simulink model "WaterTankModel_ExternalController"  (Simulink 8.1)
settings: Solver=ode3  StartTime=0.0  StopTime=150.0  FixedStep=0.001  RelTol=1e-3
InitFcn:
  | initparametersDACADC
  | WT_SerialCom_Model
undefined symbols (not defined in the file): Ad, Bd, Cd, Dd, k0, k1, k2, SAMPLING_PERIOD, WT_CALIBRATION, x0, x_ref
libraries: GisooLib x7
settings Model: Creator=behdad  LastModifiedBy=behdad

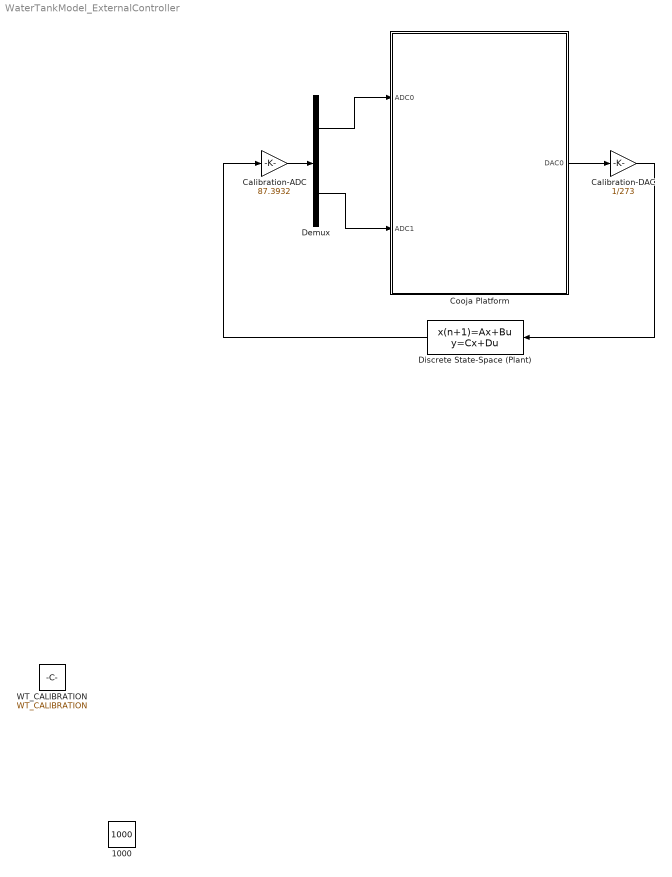
== system WaterTankModel_ExternalController ==
  1000 : Constant  Value=1000
  Calibration-ADC : Gain  Gain=87.3932
  Calibration-DAC : Gain  Gain=1/273
  Cooja Platform : Subsystem  AncestorBlock=GisooLib/Gisoo Platform  TreatAsAtomicUnit=on
  Demux : Demux  Outputs=2
  Discrete State-Space (Plant) : DiscreteStateSpace  A=Ad  B=Bd  C=Cd  D=Dd  X0=x0  SampleTime=-1
  WT_CALIBRATION : Constant  Value=WT_CALIBRATION
  wires:
  Discrete State-Space (Plant)/1 -> Calibration-ADC/1
  Cooja Platform/1(DAC0) -> Calibration-DAC/1
  Calibration-DAC/1 -> Discrete State-Space (Plant)/1
  Calibration-ADC/1 -> Demux/1
  Demux/1 -> Cooja Platform/1(ADC0)
  Demux/2 -> Cooja Platform/2(ADC1)

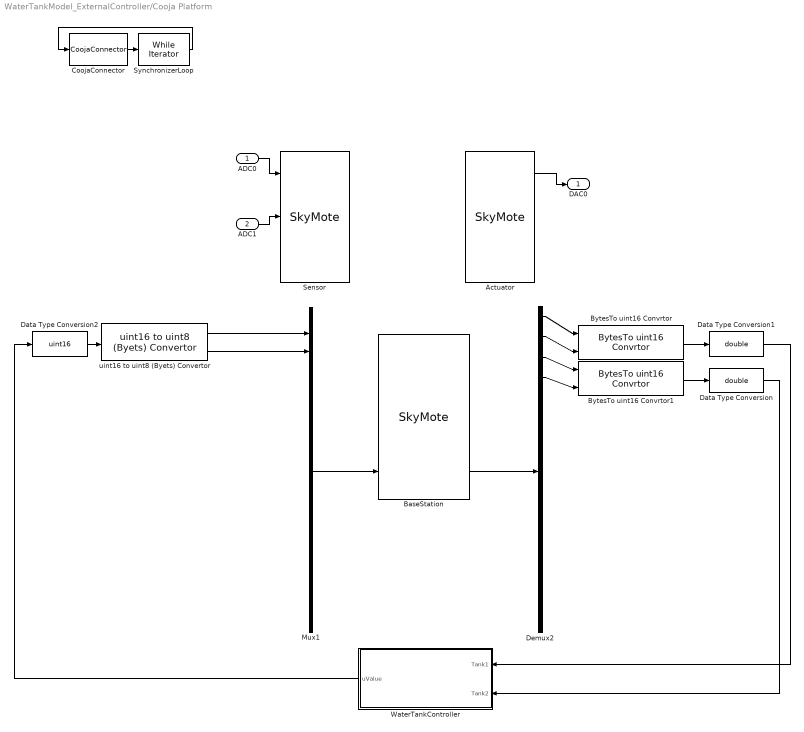
== system WaterTankModel_ExternalController/Cooja Platform ==
  ADC0 : Inport
  ADC1 : Inport  Port=2
  Actuator : GisooLib/SkyMote  moteID=4  PacketType=6
  BaseStation : GisooLib/SkyMote  moteID=3  PacketType=6
  BytesTo uint16 Convrtor : GisooLib/BytesTo uint16 Convrtor
  BytesTo uint16 Convrtor1 : GisooLib/BytesTo uint16 Convrtor
  CoojaConnector : GisooLib/Cooja Platform/CoojaConnector
      link override "Check that we don't loop forever, if Cooja never answers": const=30000
  Data Type Conversion : DataTypeConversion  OutDataTypeStr=double
  Data Type Conversion1 : DataTypeConversion  OutDataTypeStr=double
  Data Type Conversion2 : DataTypeConversion  OutDataTypeStr=uint16
  Demux2 : Demux  Outputs=16
  Mux1 : Mux  Inputs=16
  Sensor : GisooLib/SkyMote  moteID=1  PacketType=6
  SynchronizerLoop : WhileIterator  MaxIters=-1  WhileBlockType=do-while  ShowIterationPort=on
  WaterTankController : Subsystem
  uint16 to uint8 (Byets) Convertor : GisooLib/uint16 to uint8 (Byets) Convertor
  DAC0 : Outport
  wires:
  Actuator/1 -> DAC0/1
  ADC0/1 -> Sensor/1
  ADC1/1 -> Sensor/2
  SynchronizerLoop/1 -> CoojaConnector/1
  CoojaConnector/1 -> SynchronizerLoop/1
  BaseStation/3 -> Demux2/1
  Mux1/1 -> BaseStation/3
  uint16 to uint8 (Byets) Convertor/1 -> Mux1/1
  uint16 to uint8 (Byets) Convertor/2 -> Mux1/2
  Demux2/1 -> BytesTo uint16 Convrtor/1
  Demux2/2 -> BytesTo uint16 Convrtor/2
  BytesTo uint16 Convrtor/1 -> Data Type Conversion1/1
  BytesTo uint16 Convrtor1/1 -> Data Type Conversion/1
  Data Type Conversion2/1 -> uint16 to uint8 (Byets) Convertor/1
  Data Type Conversion/1 -> WaterTankController/2(Tank2)
  WaterTankController/1(uValue) -> Data Type Conversion2/1
  Demux2/3 -> BytesTo uint16 Convrtor1/1
  Demux2/4 -> BytesTo uint16 Convrtor1/2
  Data Type Conversion1/1 -> WaterTankController/1(Tank1)

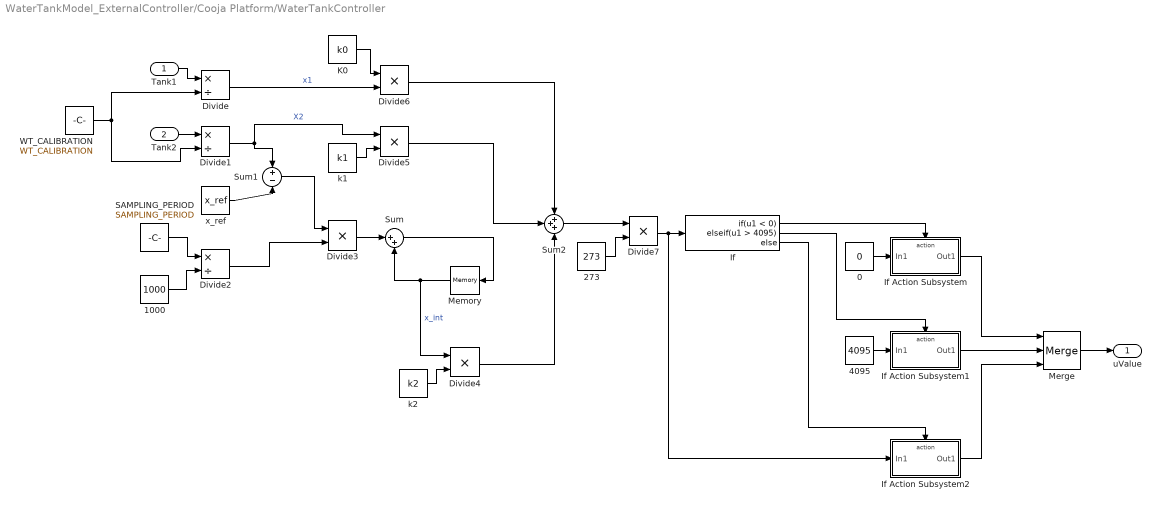
== system WaterTankModel_ExternalController/Cooja Platform/WaterTankController ==
  Tank1 : Inport
  Tank2 : Inport  Port=2
  0 : Constant  Value=0
  1000 : Constant  Value=1000
  273 : Constant  Value=273
  4095 : Constant  Value=4095
  Divide : Product  Inputs=*/
  Divide1 : Product  Inputs=*/
  Divide2 : Product  Inputs=*/
  Divide{3..7} (5 alike) : Product  Inputs=**
  If : If  IfExpression=u1 < 0  ElseIfExpressions=u1 > 4095
  If Action Subsystem : Subsystem  TreatAsAtomicUnit=on
  If Action Subsystem1 : Subsystem  TreatAsAtomicUnit=on
  If Action Subsystem2 : Subsystem  TreatAsAtomicUnit=on
  K0 : Constant  Value=k0
  Memory : Memory  InheritSampleTime=on
  Merge : Merge  Inputs=3
  SAMPLING_PERIOD : Constant  Value=SAMPLING_PERIOD
  Sum : Sum  Inputs=|++
  Sum1 : Sum  Inputs=+-
  Sum2 : Sum  Inputs=+++
  WT_CALIBRATION : Constant  Value=WT_CALIBRATION
  k1 : Constant  Value=k1
  k2 : Constant  Value=k2
  x_ref : Constant  Value=x_ref
  uValue : Outport
  wires:
  If Action Subsystem/1(Out1) -> Merge/1
  Divide5/1 -> Sum2/2
  0/1 -> If Action Subsystem/1(In1)
  1000/1 -> Divide2/2
  Divide2/1 -> Divide3/2
  x_ref/1 -> Sum1/2
  k1/1 -> Divide5/2
  Tank2/1 -> Divide1/1
  Divide1/1 -> Divide5/1, Sum1/1  "X2"
  Divide3/1 -> Sum/1
  Memory/1 -> Sum/2, Divide4/1  "x_int"
  WT_CALIBRATION/1 -> Divide/2, Divide1/2
  Divide/1 -> Divide6/2  "x1"
  k2/1 -> Divide4/2
  Tank1/1 -> Divide/1
  Divide6/1 -> Sum2/1
  If Action Subsystem2/1(Out1) -> Merge/3
  4095/1 -> If Action Subsystem1/1(In1)
  Sum2/1 -> Divide7/1
  Divide7/1 -> If/1, If Action Subsystem2/1(In1)
  If/3 -> If Action Subsystem2/Action
  If/1 -> If Action Subsystem/Action
  If Action Subsystem1/1(Out1) -> Merge/2
  Merge/1 -> uValue/1
  273/1 -> Divide7/2
  If/2 -> If Action Subsystem1/Action
  Sum/1 -> Memory/1
  Sum1/1 -> Divide3/1
  K0/1 -> Divide6/1
  Divide4/1 -> Sum2/3
  SAMPLING_PERIOD/1 -> Divide2/1

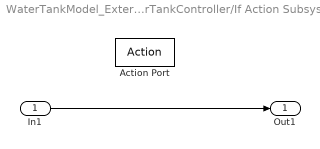
== system WaterTankModel_ExternalController/Cooja Platform/WaterTankController/If Action Subsystem ==
  In1 : Inport
  Action Port : ActionPort  ActionType=then
  Out1 : Outport
  wires:
  In1/1 -> Out1/1

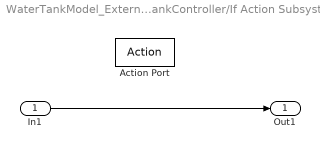
== system WaterTankModel_ExternalController/Cooja Platform/WaterTankController/If Action Subsystem1 ==
  In1 : Inport
  Action Port : ActionPort  ActionType=elseif
  Out1 : Outport
  wires:
  In1/1 -> Out1/1

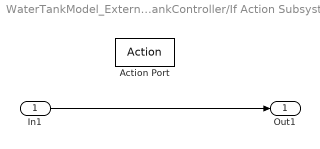
== system WaterTankModel_ExternalController/Cooja Platform/WaterTankController/If Action Subsystem2 ==
  In1 : Inport
  Action Port : ActionPort  ActionType=else
  Out1 : Outport
  wires:
  In1/1 -> Out1/1
